simulink model "RosBag_test_odometry"  (R2021a)
settings: Solver=FixedStepAuto  StartTime=0.0  StopTime=500  RelTol=1e-3
model workspace (MAT data in the model file):
  Logfile_Data_Object = robotics.ros.BagSelection
  Logfile_Data_Object.FilePath = 'C:\Users\user\Desktop\Lab-Epson 2021-12-22-10-15-22.bag'
  Logfile_Data_Object.StartTime = 1640196922.65
  Logfile_Data_Object.EndTime = 1640197404.88
  Logfile_Data_Object.NumMessages = 59577
  Logfile_Data_Object.AvailableTopics = table
  Logfile_Data_Object.AvailableTopics.data{1} = [1; 4820; 4820; 10220; 1; 1; 1; 4822; 4820; 4822; 10220; 10208; 4821]
  Logfile_Data_Object.AvailableTopics.data{2} = categorical
  Logfile_Data_Object.AvailableTopics.data{2}.categoryNames = {'dynamic_reconfigure/Config'; 'dynamic_reconfigure/ConfigDescription'; 'geometry_msgs/Twist'; 'nav_msgs/Odometry'; 'rosaria/BumperState'; 'rosgraph_msgs/Log'; 'sensor_msgs/PointCloud'; 'sensor_msgs/PointCloud2'; 'std_msgs/Bool'; 'std_msgs/Float64'; 'std_msgs/Int8'; 'tf2_msgs/TFMessage'}
  Logfile_Data_Object.AvailableTopics.data{2}.codes = [11; 10; 5; 3; 9; 2; 1; 4; 7; 8; 6; 6; 12]
  Logfile_Data_Object.AvailableTopics.data{3}{1} = ''
  Logfile_Data_Object.AvailableTopics.data{3}{2} = ''
  Logfile_Data_Object.AvailableTopics.data{3}{3} = '  uint32 Seq
    |   Time Stamp
    |   char FrameId
    | logical[] FrontBumpers
    | logical[] RearBumpers
    | '
  Logfile_Data_Object.AvailableTopics.data{3}{4} = '  double X
    |   double Y
    |   double Z
    | geometry_msgs/Vector3 Angular
    |   double X
    |   double Y
    |   double Z
    | '
  Logfile_Data_Object.AvailableTopics.data{3}{5} = ''
  Logfile_Data_Object.AvailableTopics.data{3}{6} = '  char Name
    |   char Type
    |   dynamic_reconfigure/ParamDescription[] Parameters
    |     char Name
    |     char Type
    |     uint32 Level
    |     char Description
    |     char EditMethod
    |   int32 Parent
    |   int32 Id
    | dynamic_reconfigure/Config Max
    |   dynamic_reconfigure/BoolParameter[] Bools
    |     char Name
    |     logical Value
    |   dynamic_reconfigure/IntParameter[] Ints
    |     char Name
    |     int32 Value
    |   dynamic_reconfigure/StrParameter[] Strs
    |     char Name
    |     char Value
    |   dynamic_reconfigure/DoubleParameter[] Doubles
    |     char Name
    |     double Value
    |   dynamic_reconfigure/GroupState[] Groups
    |     char Name
    |     logical State
    |     int32 Id
    |     int32 Parent
    | dynamic_reconfigure/Config Min
    |   dynamic_reconfigure/BoolParameter[] Bools
    |     char Name
    |     logical Value
    |   dynamic_reconfigure/IntParameter[] Ints
    |     char Name
    |     int32 Value
    |   dynamic_reconfigure/StrParameter[] Strs
    |     char Name
    |     char Value
    |   dynamic_reconfigure/DoubleParameter[] Doubles
    |     char Name
    |     double Value
    |   dynamic_reconfigure/GroupState[] Groups
    |     char Name
    |     logical State
    |     int32 Id
    |     int32 Parent
    | dynamic_reconfigure/Config Dflt
    |   dynamic_reconfigure/BoolParameter[] Bools
    |     char Name
    |     logical Value
    |   dynamic_reconfigure/IntParameter[] Ints
    |     char Name
    |     int32 Value
    |   dynamic_reconfigure/StrParameter[] Strs
    |     char Name
    |     char Value
    |   dynamic_reconfigure/DoubleParameter[] Doubles
    |     char Name
    |     double Value
    |   dynamic_reconfigure/GroupState[] Groups
    |     char Name
    |     logical State
    |     int32 Id
    |     int32 Parent
    | '
  Logfile_Data_Object.AvailableTopics.data{3}{7} = '  char Name
    |   logical Value
    | dynamic_reconfigure/IntParameter[] Ints
    |   char Name
    |   int32 Value
    | dynamic_reconfigure/StrParameter[] Strs
    |   char Name
    |   char Value
    | dynamic_reconfigure/DoubleParameter[] Doubles
    |   char Name
    |   double Value
    | dynamic_reconfigure/GroupState[] Groups
    |   char Name
    |   logical State
    |   int32 Id
    |   int32 Parent
    | '
  Logfile_Data_Object.AvailableTopics.data{3}{8} = '  uint32 Seq
    |   Time Stamp
    |   char FrameId
    | char ChildFrameId
    | geometry_msgs/PoseWithCovariance Pose
    |   geometry_msgs/Pose Pose
    |     geometry_msgs/Point Position
    |       double X
    |       double Y
    |       double Z
    |     geometry_msgs/Quaternion Orientation
    |       double X
    |       double Y
    |       double Z
    |       double W
    |   double[36] Covariance
    | geometry_msgs/TwistWithCovariance Twist
    |   geometry_msgs/Twist Twist
    |     geometry_msgs/Vector3 Linear
    |       double X
    |       double Y
    |       double Z
    |     geometry_msgs/Vector3 Angular
    |       double X
    |       double Y
    |       double Z
    |   double[36] Covariance
    | '
  Logfile_Data_Object.AvailableTopics.data{3}{9} = '  uint32 Seq
    |   Time Stamp
    |   char FrameId
    | geometry_msgs/Point32[] Points
    |   single X
    |   single Y
    |   single Z
    | sensor_msgs/ChannelFloat32[] Channels
    |   char Name
    |   single[] Values
    | '
  Logfile_Data_Object.AvailableTopics.data{3}{10} = '  uint32 Seq
    |   Time Stamp
    |   char FrameId
    | uint32 Height
    | uint32 Width
    | sensor_msgs/PointField[] Fields
    |   uint8 INT8
    |   uint8 UINT8
    |   uint8 INT16
    |   uint8 UINT16
    |   uint8 INT32
    |   uint8 UINT32
    |   uint8 FLOAT32
    |   uint8 FLOAT64
    |   char Name
    |   uint32 Offset
    |   uint8 Datatype
    |   uint32 Count
    | logical IsBigendian
    | uint32 PointStep
    | uint32 RowStep
    | uint8[] Data
    | logical IsDense
    | '
  Logfile_Data_Object.AvailableTopics.data{3}{11} = 'int8 INFO
    | int8 WARN
    | int8 ERROR
    | int8 FATAL
    | std_msgs/Header Header
    |   uint32 Seq
    |   Time Stamp
    |   char FrameId
    | int8 Level
    | char Name
    | char Msg
    | char File
    | char Function
    | uint32 Line
    | char[] Topics
    | '
  Logfile_Data_Object.AvailableTopics.data{3}{12} = 'int8 INFO
    | int8 WARN
    | int8 ERROR
    | int8 FATAL
    | std_msgs/Header Header
    |   uint32 Seq
    |   Time Stamp
    |   char FrameId
    | int8 Level
    | char Name
    | char Msg
    | char File
    | char Function
    | uint32 Line
    | char[] Topics
    | '
  Logfile_Data_Object.AvailableTopics.data{3}{13} = '  std_msgs/Header Header
    |     uint32 Seq
    |     Time Stamp
    |     char FrameId
    |   char ChildFrameId
    |   geometry_msgs/Transform Transform
    |     geometry_msgs/Vector3 Translation
    |       double X
    |       double Y
    |       double Z
    |     geometry_msgs/Quaternion Rotation
    |       double X
    |       double Y
    |       double Z
    |       double W
    | '
  Logfile_Data_Object.AvailableTopics.ndims = 2
  Logfile_Data_Object.AvailableTopics.nrows = 13
  Logfile_Data_Object.AvailableTopics.rownames = {'/RosAria/battery_recharge_state'; '/RosAria/battery_voltage'; '/RosAria/bumper_state'; '/RosAria/cmd_vel'; '/RosAria/motors_state'; '/RosAria/parameter_descriptions'; '/RosAria/parameter_updates'; '/RosAria/pose'; '/RosAria/sonar'; '/RosAria/sonar_pointcloud2'; '/rosout'; '/rosout_agg'; '/tf'}
  Logfile_Data_Object.AvailableTopics.nvars = 3
  Logfile_Data_Object.AvailableTopics.varnames = {'NumMessages', 'MessageType', 'MessageDefinition'}
  Logfile_Data_Object.AvailableTopics.props.useVariableNamesOriginal = 0
  Logfile_Data_Object.AvailableTopics.props.useDimensionNamesOriginal = 0
  Logfile_Data_Object.AvailableTopics.props.CustomProps = struct()
  Logfile_Data_Object.AvailableTopics.props.VariableCustomProps = struct()
  Logfile_Data_Object.AvailableTopics.props.versionSavedFrom = 4
  Logfile_Data_Object.AvailableTopics.props.minCompatibleVersion = 1
  Logfile_Data_Object.AvailableTopics.props.incompatibilityMsg = ''
  Logfile_Data_Object.AvailableTopics.props.VersionSavedFrom = 4
  Logfile_Data_Object.AvailableTopics.props.Description = ''
  Logfile_Data_Object.AvailableTopics.props.VariableNamesOriginal = {}
  Logfile_Data_Object.AvailableTopics.props.DimensionNames = {'Row', 'Variables'}
  Logfile_Data_Object.AvailableTopics.props.DimensionNamesOriginal = {}
  Logfile_Data_Object.AvailableTopics.props.UserData = []
  Logfile_Data_Object.AvailableTopics.props.VariableDescriptions = {}
  Logfile_Data_Object.AvailableTopics.props.VariableUnits = {}
  Logfile_Data_Object.AvailableTopics.props.VariableContinuity = {}
  Logfile_Data_Object.AvailableFrames = {'base_link'; 'odom'}
  Logfile_Data_Object.MessageList = table
  Logfile_Data_Object.MessageList.data{1} = [1640196922.65 1640196922.65 1640196922.65 1640196922.65 1640196922.65 1640196922.65 1640196922.65 1640196922.65 1640196922.65 1640196922.65 1640196922.67 1640196922.67 ... (59577 elements, 59577x1)]
  Logfile_Data_Object.MessageList.data{2} = categorical
  Logfile_Data_Object.MessageList.data{2}.categoryNames = {'/RosAria/battery_recharge_state'; '/RosAria/battery_voltage'; '/RosAria/bumper_state'; '/RosAria/cmd_vel'; '/RosAria/motors_state'; '/RosAria/parameter_descriptions'; '/RosAria/parameter_updates'; '/RosAria/pose'; '/RosAria/sonar'; '/RosAria/sonar_pointcloud2'; '/rosout'; '/rosout_agg'; '/tf'}
  Logfile_Data_Object.MessageList.data{2}.codes = [11 11 11 11 11 11 11 11 11 11 6 5 ... (59577 elements, 59577x1)]
  Logfile_Data_Object.MessageList.data{3} = categorical
  Logfile_Data_Object.MessageList.data{3}.categoryNames = {'std_msgs/Int8'; 'std_msgs/Float64'; 'rosaria/BumperState'; 'geometry_msgs/Twist'; 'std_msgs/Bool'; 'dynamic_reconfigure/ConfigDescription'; 'dynamic_reconfigure/Config'; 'nav_msgs/Odometry'; 'sensor_msgs/PointCloud'; 'sensor_msgs/PointCloud2'; 'rosgraph_msgs/Log'; 'tf2_msgs/TFMessage'}
  Logfile_Data_Object.MessageList.data{3}.codes = [11 11 11 11 11 11 11 11 11 11 6 5 ... (59577 elements, 59577x1)]
  Logfile_Data_Object.MessageList.data{4} = [5486 5746 6002 6281 6566 6840 7104 7381 7665 7932 9864 11694 ... (59577 elements, 59577x1)]
  Logfile_Data_Object.MessageList.ndims = 2
  Logfile_Data_Object.MessageList.nrows = 59577
  Logfile_Data_Object.MessageList.nvars = 4
  Logfile_Data_Object.MessageList.varnames = {'Time', 'Topic', 'MessageType', 'FileOffset'}
  Logfile_Data_Object.MessageList.props.useVariableNamesOriginal = 0
  Logfile_Data_Object.MessageList.props.useDimensionNamesOriginal = 0
  Logfile_Data_Object.MessageList.props.CustomProps = struct()
  Logfile_Data_Object.MessageList.props.VariableCustomProps = struct()
  Logfile_Data_Object.MessageList.props.versionSavedFrom = 4
  Logfile_Data_Object.MessageList.props.minCompatibleVersion = 1
  Logfile_Data_Object.MessageList.props.incompatibilityMsg = ''
  Logfile_Data_Object.MessageList.props.VersionSavedFrom = 4
  Logfile_Data_Object.MessageList.props.Description = ''
  Logfile_Data_Object.MessageList.props.VariableNamesOriginal = {}
  Logfile_Data_Object.MessageList.props.DimensionNames = {'Row', 'Variables'}
  Logfile_Data_Object.MessageList.props.DimensionNamesOriginal = {}
  Logfile_Data_Object.MessageList.props.UserData = []
  Logfile_Data_Object.MessageList.props.VariableDescriptions = {}
  Logfile_Data_Object.MessageList.props.VariableUnits = {}
  Logfile_Data_Object.MessageList.props.VariableContinuity = {}
  Logfile_Data_Object.TopicTypeMap = containers.Map
  Logfile_Data_Object.TopicTypeMap.serialization.keys = {'/RosAria/battery_recharge_state', '/RosAria/battery_voltage', '/RosAria/bumper_state', '/RosAria/cmd_vel', '/RosAria/motors_state', '/RosAria/parameter_descriptions', '/RosAria/parameter_updates', '/RosAria/pose', '/RosAria/sonar', '/RosAria/sonar_pointcloud2', '/rosout', '/rosout_agg', '/tf'}
  Logfile_Data_Object.TopicTypeMap.serialization.values = {'std_msgs/Int8', 'std_msgs/Float64', 'rosaria/BumperState', 'geometry_msgs/Twist', 'std_msgs/Bool', 'dynamic_reconfigure/ConfigDescription', 'dynamic_reconfigure/Config', 'nav_msgs/Odometry', 'sensor_msgs/PointCloud', 'sensor_msgs/PointCloud2', 'rosgraph_msgs/Log', 'rosgraph_msgs/Log', 'tf2_msgs/TFMessage'}
  Logfile_Data_Object.TopicTypeMap.serialization.uniformity = 1
  Logfile_Data_Object.TopicTypeMap.serialization.keyType = 'char'
  Logfile_Data_Object.TopicTypeMap.serialization.valueType = 'char'
  Logfile_Data_Object.TopicDefinitionMap = containers.Map
  Logfile_Data_Object.TopicDefinitionMap.serialization.keys = {'/RosAria/battery_recharge_state', '/RosAria/battery_voltage', '/RosAria/bumper_state', '/RosAria/cmd_vel', '/RosAria/motors_state', '/RosAria/parameter_descriptions', '/RosAria/parameter_updates', '/RosAria/pose', '/RosAria/sonar', '/RosAria/sonar_pointcloud2', '/rosout', '/rosout_agg', '/tf'}
  Logfile_Data_Object.TopicDefinitionMap.serialization.values{1} = ''
  Logfile_Data_Object.TopicDefinitionMap.serialization.values{2} = ''
  Logfile_Data_Object.TopicDefinitionMap.serialization.values{3} = '  uint32 Seq
    |   Time Stamp
    |   char FrameId
    | logical[] FrontBumpers
    | logical[] RearBumpers
    | '
  Logfile_Data_Object.TopicDefinitionMap.serialization.values{4} = '  double X
    |   double Y
    |   double Z
    | geometry_msgs/Vector3 Angular
    |   double X
    |   double Y
    |   double Z
    | '
  Logfile_Data_Object.TopicDefinitionMap.serialization.values{5} = ''
  Logfile_Data_Object.TopicDefinitionMap.serialization.values{6} = '  char Name
    |   char Type
    |   dynamic_reconfigure/ParamDescription[] Parameters
    |     char Name
    |     char Type
    |     uint32 Level
    |     char Description
    |     char EditMethod
    |   int32 Parent
    |   int32 Id
    | dynamic_reconfigure/Config Max
    |   dynamic_reconfigure/BoolParameter[] Bools
    |     char Name
    |     logical Value
    |   dynamic_reconfigure/IntParameter[] Ints
    |     char Name
    |     int32 Value
    |   dynamic_reconfigure/StrParameter[] Strs
    |     char Name
    |     char Value
    |   dynamic_reconfigure/DoubleParameter[] Doubles
    |     char Name
    |     double Value
    |   dynamic_reconfigure/GroupState[] Groups
    |     char Name
    |     logical State
    |     int32 Id
    |     int32 Parent
    | dynamic_reconfigure/Config Min
    |   dynamic_reconfigure/BoolParameter[] Bools
    |     char Name
    |     logical Value
    |   dynamic_reconfigure/IntParameter[] Ints
    |     char Name
    |     int32 Value
    |   dynamic_reconfigure/StrParameter[] Strs
    |     char Name
    |     char Value
    |   dynamic_reconfigure/DoubleParameter[] Doubles
    |     char Name
    |     double Value
    |   dynamic_reconfigure/GroupState[] Groups
    |     char Name
    |     logical State
    |     int32 Id
    |     int32 Parent
    | dynamic_reconfigure/Config Dflt
    |   dynamic_reconfigure/BoolParameter[] Bools
    |     char Name
    |     logical Value
    |   dynamic_reconfigure/IntParameter[] Ints
    |     char Name
    |     int32 Value
    |   dynamic_reconfigure/StrParameter[] Strs
    |     char Name
    |     char Value
    |   dynamic_reconfigure/DoubleParameter[] Doubles
    |     char Name
    |     double Value
    |   dynamic_reconfigure/GroupState[] Groups
    |     char Name
    |     logical State
    |     int32 Id
    |     int32 Parent
    | '
  Logfile_Data_Object.TopicDefinitionMap.serialization.values{7} = '  char Name
    |   logical Value
    | dynamic_reconfigure/IntParameter[] Ints
    |   char Name
    |   int32 Value
    | dynamic_reconfigure/StrParameter[] Strs
    |   char Name
    |   char Value
    | dynamic_reconfigure/DoubleParameter[] Doubles
    |   char Name
    |   double Value
    | dynamic_reconfigure/GroupState[] Groups
    |   char Name
    |   logical State
    |   int32 Id
    |   int32 Parent
    | '
  Logfile_Data_Object.TopicDefinitionMap.serialization.values{8} = '  uint32 Seq
    |   Time Stamp
    |   char FrameId
    | char ChildFrameId
    | geometry_msgs/PoseWithCovariance Pose
    |   geometry_msgs/Pose Pose
    |     geometry_msgs/Point Position
    |       double X
    |       double Y
    |       double Z
    |     geometry_msgs/Quaternion Orientation
    |       double X
    |       double Y
    |       double Z
    |       double W
    |   double[36] Covariance
    | geometry_msgs/TwistWithCovariance Twist
    |   geometry_msgs/Twist Twist
    |     geometry_msgs/Vector3 Linear
    |       double X
    |       double Y
    |       double Z
    |     geometry_msgs/Vector3 Angular
    |       double X
    |       double Y
    |       double Z
    |   double[36] Covariance
    | '
  Logfile_Data_Object.TopicDefinitionMap.serialization.values{9} = '  uint32 Seq
    |   Time Stamp
    |   char FrameId
    | geometry_msgs/Point32[] Points
    |   single X
    |   single Y
    |   single Z
    | sensor_msgs/ChannelFloat32[] Channels
    |   char Name
    |   single[] Values
    | '
  Logfile_Data_Object.TopicDefinitionMap.serialization.values{10} = '  uint32 Seq
    |   Time Stamp
    |   char FrameId
    | uint32 Height
    | uint32 Width
    | sensor_msgs/PointField[] Fields
    |   uint8 INT8
    |   uint8 UINT8
    |   uint8 INT16
    |   uint8 UINT16
    |   uint8 INT32
    |   uint8 UINT32
    |   uint8 FLOAT32
    |   uint8 FLOAT64
    |   char Name
    |   uint32 Offset
    |   uint8 Datatype
    |   uint32 Count
    | logical IsBigendian
    | uint32 PointStep
    | uint32 RowStep
    | uint8[] Data
    | logical IsDense
    | '
  Logfile_Data_Object.TopicDefinitionMap.serialization.values{11} = 'int8 INFO
    | int8 WARN
    | int8 ERROR
    | int8 FATAL
    | std_msgs/Header Header
    |   uint32 Seq
    |   Time Stamp
    |   char FrameId
    | int8 Level
    | char Name
    | char Msg
    | char File
    | char Function
    | uint32 Line
    | char[] Topics
    | '
  Logfile_Data_Object.TopicDefinitionMap.serialization.values{12} = 'int8 INFO
    | int8 WARN
    | int8 ERROR
    | int8 FATAL
    | std_msgs/Header Header
    |   uint32 Seq
    |   Time Stamp
    |   char FrameId
    | int8 Level
    | char Name
    | char Msg
    | char File
    | char Function
    | uint32 Line
    | char[] Topics
    | '
  Logfile_Data_Object.TopicDefinitionMap.serialization.values{13} = '  std_msgs/Header Header
    |     uint32 Seq
    |     Time Stamp
    |     char FrameId
    |   char ChildFrameId
    |   geometry_msgs/Transform Transform
    |     geometry_msgs/Vector3 Translation
    |       double X
    |       double Y
    |       double Z
    |     geometry_msgs/Quaternion Rotation
    |       double X
    |       double Y
    |       double Z
    |       double W
    | '
  Logfile_Data_Object.TopicDefinitionMap.serialization.uniformity = 1
  Logfile_Data_Object.TopicDefinitionMap.serialization.keyType = 'char'
  Logfile_Data_Object.TopicDefinitionMap.serialization.valueType = 'char'
  Logfile_Data_Object.messageTypeMap = containers.Map
  Logfile_Data_Object.messageTypeMap.serialization.keys = {}
  Logfile_Data_Object.messageTypeMap.serialization.values = {}
  Logfile_Data_Object.messageTypeMap.serialization.uniformity = 0
  Logfile_Data_Object.messageTypeMap.serialization.keyType = 'char'
  Logfile_Data_Object.messageTypeMap.serialization.valueType = 'any'
  Logfile_Data_Object.Parser = robotics.ros.internal.tf.TransformationTreeParser
  Logfile_Data_Object.Parser.UseObjectMsg = 1
  Logfile_Path = 'C:\Users\user\Desktop\Lab-Epson 2021-12-22-10-15-22.bag'
  Logfile_Playback_Duration = nan
  Logfile_Playback_Offset = nan
libraries: robotcorelib x1, robotlib x1, simulink x1
settings Model: Creator=user  LastModifiedBy=user
settings SolverCC: AlgebraicLoopSolver=TrustRegion
settings OptimizationCC: EnhancedBackFolding=on  PassReuseOutputArgsAs=Individual arguments  ZeroExternalMemoryAtStartup=off  ZeroInternalMemoryAtStartup=off  MaxStackSize=64  OptimizeBlockOrder=speed  DifferentSizesBufferReuse=on  OptimizationCustomize=off  EfficientTunableParamExpr=on
settings DebuggingCC: ParameterTunabilityLossMsg=error  SFMachineParentedDataDiag=warning
settings HardwareCC: ProdBitPerPointer=32  ProdBitPerSizeT=32  ProdBitPerPtrDiffT=32  ProdLargestAtomicFloat=None  ProdIntDivRoundTo=Undefined  ProdEndianess=Unspecified  ProdWordSize=32  ProdHWDeviceType=Generic->Unspecified (assume 32-bit Generic)
settings SFSimCC: MATLABDynamicMemAlloc=off  SimTargetLang=C++
settings RTWCC: SystemTargetFile=ert.tlc  HardwareBoard=Robot Operating System (ROS)  TLCOptions="-aInlineSetEventsForThisBaseRateFcn=TLC_FALSE -aSuppressMultiTaskScheduler=TLC_FALSE  -aRateBasedStepFcn=0"  TemplateMakefile=ert_default_tmf  Toolchain=Catkin  TargetLang=C++
settings CodeAppCC: ForceParamTrailComments=on  IgnoreCustomStorageClasses=off  OperatorAnnotations=on  SimulinkDataObjDesc=on  SFDataObjDesc=on  InsertBlockDesc=on

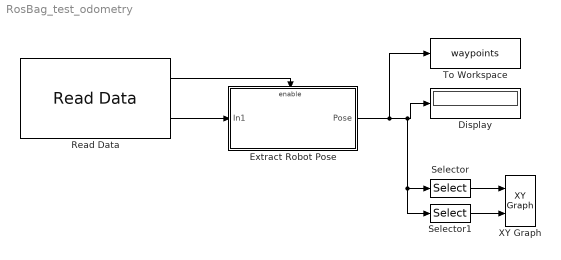
== system RosBag_test_odometry ==
  Display : Display
  Extract Robot Pose : Subsystem
  Read Data : robotlib/Read Data  topic=/RosAria/pose  sampleTime=-1  logfileType=rosbag  modelName=RosBag_test_odometry  msgType=nav_msgs/Odometry
      settings: SourceProductBaseCode=RR
  Selector : Selector  InputPortWidth=3  IndexOptions=Index vector (dialog)  Indices=[1]  OutputSizes=1
  Selector1 : Selector  InputPortWidth=3  IndexOptions=Index vector (dialog)  Indices=[2]  OutputSizes=1
  To Workspace : ToWorkspace  VariableName=waypoints  SampleTime=1
      settings: Save2DSignal=2-D array (concatenate along first dimension)
  XY Graph : simulink/Sinks/XY Graph  xmin=0  xmax=35  ymin=0  ymax=25  st=1
  wires:
  Read Data/2 -> Extract Robot Pose/1(In1)
  Read Data/1 -> Extract Robot Pose/Enable
  Selector1/1 -> XY Graph/2
  Extract Robot Pose/1(Pose) -> To Workspace/1, Selector/1, Selector1/1, Display/1
  Selector/1 -> XY Graph/1

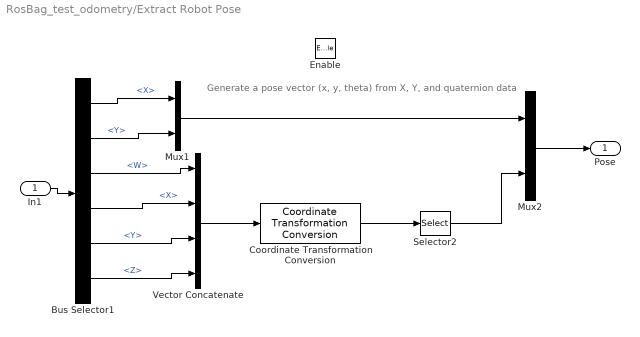
== system RosBag_test_odometry/Extract Robot Pose ==
  note: Generate a pose vector (x, y, theta) from X, Y, and quaternion data
  In1 : Inport
  Enable : EnablePort
  Bus Selector1 : BusSelector  OutputSignals=Pose.Pose.Position.X,Pose.Pose.Position.Y,Pose.Pose.Orientation.W,Pose.Pose.Orientation.X,Pose.Pose.Orientation.Y,Pose.Pose.Orientation.Z
  Coordinate Transformation Conversion : robotcorelib/Coordinate Transformation Conversion  InputRepresentation=Quaternion  InputEulerSequence=ZYX  ShowTrVecInputPort=on  OutputRepresentation=Euler Angles  OutputEulerSequence=ZYX  ShowTrVecOutputPort=on  SimulateUsing=Interpreted execution
      settings: SourceProductBaseCode=NV,RO,RR,UV
  Mux1 : Mux  Inputs=2
  Mux2 : Mux  Inputs=2
  Selector2 : Selector  InputPortWidth=3  IndexOptions=Index vector (dialog)  Indices=1  OutputSizes=1
  Vector Concatenate : Concatenate  NumInputs=4
  Pose : Outport  VectorParamsAs1DForOutWhenUnconnected=off
  wires:
  Vector Concatenate/1 -> Coordinate Transformation Conversion/1
  Coordinate Transformation Conversion/1 -> Selector2/1
  Mux1/1 -> Mux2/1
  Selector2/1 -> Mux2/2
  Mux2/1 -> Pose/1
  Bus Selector1/6 -> Vector Concatenate/4  "<Z>"
  Bus Selector1/1 -> Mux1/1  "<X>"
  Bus Selector1/4 -> Vector Concatenate/2  "<X>"
  Bus Selector1/2 -> Mux1/2  "<Y>"
  Bus Selector1/5 -> Vector Concatenate/3  "<Y>"
  In1/1 -> Bus Selector1/1
  Bus Selector1/3 -> Vector Concatenate/1  "<W>"
